simulink model "curtain"  (R2018b)
settings: Solver=VariableStepAuto  StartTime=0.0  StopTime=10.0  RelTol=1e-3
model workspace (MATLAB code in the model file):
  | r_r=20e-3; %Radius of roller
  | a=5; % Height of curtain
  | b=4; % Width of curtain
  | c=1e-3; % Thickness of
  | g=9.8;
  | m_r=10; %mass of inner roller
  | m_w = 25/2*b; % mass of counter weights
  | f_c=1; %N/(m/s)/m friction of hanging curtain
  | f_r=0.1; %Nm/(rad/s) friction of roller
  | rho=1300 %kg/(m3) density of PVC
settings Model: Creator=kjartan  LastModifiedBy=kjartan

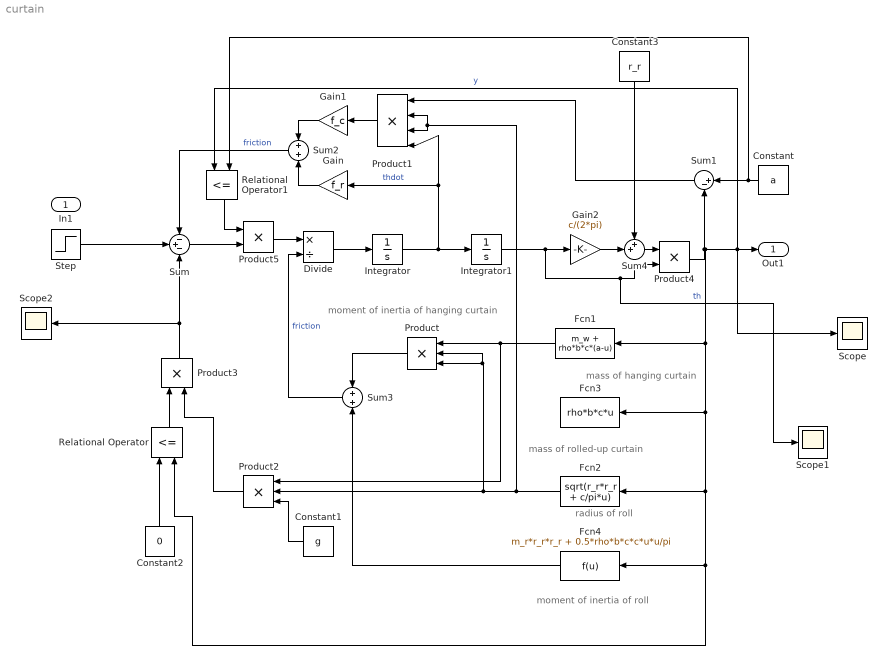
== system curtain ==
  note: moment of inertia of hanging curtain
  note: moment of inertia of roll
  note: mass of rolled-up curtain
  note: radius of roll
  note: mass of hanging curtain
  In1 : Inport
  Constant : Constant  Value=a
  Constant1 : Constant  Value=g
  Constant2 : Constant  Value=0
  Constant3 : Constant  Value=r_r
  Divide : Product  Inputs=*/
  Fcn1 : Fcn  Expr=m_w + rho*b*c*(a-u)
  Fcn2 : Fcn  Expr=sqrt(r_r*r_r + c/pi*u)
  Fcn3 : Fcn  Expr=rho*b*c*u
  Fcn4 : Fcn  Expr=m_r*r_r*r_r + 0.5*rho*b*c*c*u*u/pi
  Gain : Gain  Gain=f_r
  Gain1 : Gain  Gain=f_c
  Gain2 : Gain  Gain=c/(2*pi)
  Integrator : Integrator
  Integrator1 : Integrator  InitialCondition=12*2*pi
  Product : Product  Inputs=3
  Product1 : Product  Inputs=4
  Product2 : Product  Inputs=3
  Product3 : Product
  Product4 : Product
  Product5 : Product
  Relational Operator : RelationalOperator  Operator=<=  OutDataTypeStr=boolean  RndMeth=Simplest
  Relational Operator1 : RelationalOperator  Operator=<=  OutDataTypeStr=boolean  RndMeth=Simplest
  Scope : Scope
  Scope1 : Scope
  Scope2 : Scope
  Step : Step  Time=2  After=0  SampleTime=0
  Sum : Sum  Inputs=-+-
  Sum1 : Sum  Inputs=|+-
  Sum2 : Sum  Inputs=+|+
  Sum3 : Sum  Inputs=+|+
  Sum4 : Sum  Inputs=++|
  Out1 : Outport
  wires:
  Integrator/1 -> Product1/4, Gain/1, Integrator1/1  "thdot"
  Integrator1/1 -> Scope1/1, Product4/2, Gain2/1  "th"
  Product4/1 -> Relational Operator/2, Fcn4/1, Fcn2/1, Fcn3/1, Fcn1/1, Relational Operator1/1, Scope/1, Out1/1, Sum1/2  "y"
  Fcn1/1 -> Product2/1, Product/1
  Fcn2/1 -> Product1/2, Product1/3, Product2/2, Product/2, Product/3
  Constant/1 -> Relational Operator1/2, Sum1/1
  Sum1/1 -> Product1/1
  Product1/1 -> Gain1/1
  Gain1/1 -> Sum2/1
  Gain/1 -> Sum2/2
  Sum2/1 -> Sum/1  "friction"
  Divide/1 -> Integrator/1
  Product/1 -> Sum3/1
  Fcn4/1 -> Sum3/2
  Sum3/1 -> Divide/2  "friction"
  Constant1/1 -> Product2/3
  Constant2/1 -> Relational Operator/1
  Relational Operator/1 -> Product3/1
  Product2/1 -> Product3/2
  Product3/1 -> Sum/3, Scope2/1
  Gain2/1 -> Sum4/2
  Constant3/1 -> Sum4/1
  Sum4/1 -> Product4/1
  Product5/1 -> Divide/1
  Sum/1 -> Product5/2
  Relational Operator1/1 -> Product5/1
  Step/1 -> Sum/2
